simulink model "ParameterTests"  (R2019b)
settings: Solver=FixedStepAuto  StartTime=0.0  StopTime=tf  RelTol=1e-3  EnableMultiTasking=on
undefined symbols (not defined in the file or in its folder): bias
libraries: xpcrtudplib x4, slrtlib x4, xpcutilitieslib x3, speedgoatlib_IO101 x2, dspstat3 x2, dspsrcs4 x1
settings Model: SimulationMode=external  Creator=kflambet  LastModifiedBy=Sharma Lab
settings SolverCC: ConcurrentTasks=on  AutoInsertRateTranBlk=on
settings DataIOCC: SaveFormat=StructureWithTime
settings OptimizationCC: BlockReduction=off  OptimizeBlockIOStorage=off  BufferReuse=off  GlobalBufferReuse=off  ExpressionFolding=off  LocalBlockOutputs=off  OptimizeDataStoreBuffers=off  BusAssignmentInplaceUpdate=off
settings HardwareCC: ProdBitPerPointer=32  ProdBitPerSizeT=32  ProdBitPerPtrDiffT=32  ProdLargestAtomicFloat=None  ProdWordSize=32  ProdLongLongMode=on  ProdHWDeviceType=Generic->32-bit x86 compatible
settings RTWCC: Description=Simulink Real-Time  SystemTargetFile=slrt.tlc  TemplateMakefile=slrt_default_tmf  CodeExecutionProfiling=on  RTWCompilerOptimization=on
settings SimulinkRealTimeCC: SupportVariableSizeSignals=on  PreserveStateflowLocalDataDimensions=off  RL32LogTETModifier=off  xPCConcurrentTasks=on

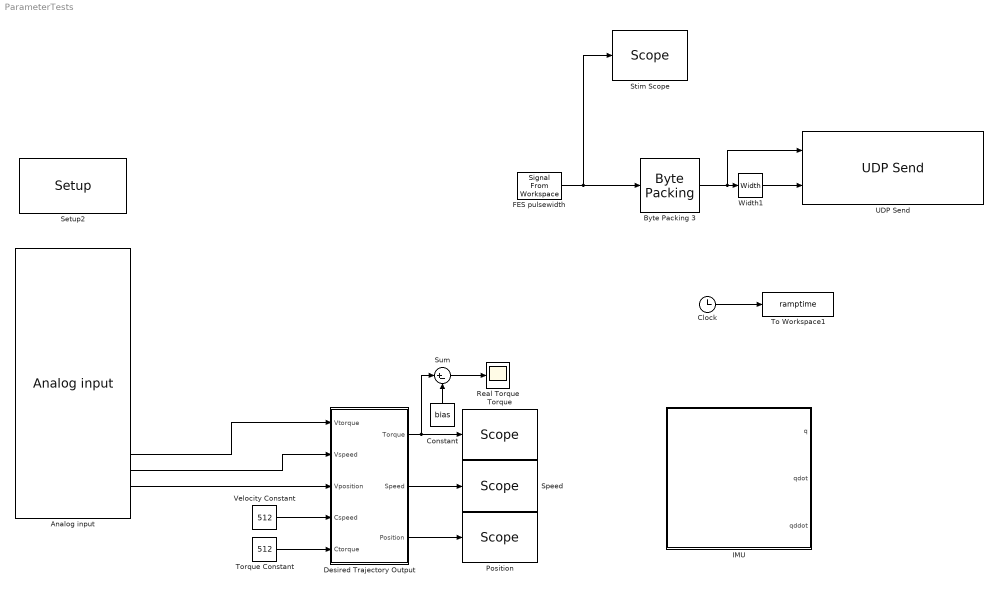
== system ParameterTests ==
  Analog input : speedgoatlib_IO101/Analog input  id=1  startChannel=1  numChannels=16  coupling=1  range=3  acqMode=1  outpMode=Values  ts=0.001  pciSlot=-1
      settings: SourceProductName=Simulink Real-Time: Speedgoat Library
  Byte Packing 3 : xpcutilitieslib/Byte Packing   MaskPackedDataType=uint8  MaskUnpackedDataTypes={ 'double'}  MaskAlignment=8
  Clock : Clock
  Constant : Constant  Value=bias
  Desired Trajectory Output : MATLAB Function  TreatAsAtomicUnit=on
  FES pulsewidth : dspsrcs4/Signal From Workspace  X=stim  Ts=0.001  nsamps=1  OutputAfterFinalValue=Setting to zero  ignoreOrWarnInputAndFrameLengths=off  OutputFrames=off
  IMU : Subsystem
  Position : slrtlib/Displays and Logging/Scope   scopeno=3  scopetype=Target  autostart=on  viewmode=Graphical sliding  formatstr='%15.6f'  grid=on  ylimits=[-360 360]  nosamples=10000  noprepostsamples=0  interleave=1  triggermode=FreeRun  triggersignal=1  trigsignalfromport=off  triggerlevel=0.0  triggerslope=Either  triggerscope=1  triggersample=0  filename=data.dat  mode=Lazy  writesize=512  autorestart=off  dynamicfilemode=off  maxwritefilesize=512*1024^2
  Real Torque : Scope
  Setup2 : speedgoatlib_IO101/Setup  group=Analog input setup  id=1  pciSlot=-1  adStartChannel=1  adNumChannel=16  adCoupling=Differential  adRange="-10 .. 10V ==> Set  hardware DIP switches 2 5 6 9 to ON"  adAcqMode=Standard  daChannel=[1:8]  daReset=[1]  daInitValue=[0]  lowerChannel=1  lowerDirection=Input  lowerDIDebounce=0  lowerDOReset=[1]  lowerDOInitValues=[0]  upperChannel=1  upperDirection=Output  upperDIDebounce=0  upperDOReset=0  upperDOInitValues=0
      settings: SourceProductName=Simulink Real-Time: Speedgoat Library
  Speed : slrtlib/Displays and Logging/Scope   scopeno=5  scopetype=Target  autostart=on  viewmode=Graphical sliding  formatstr='%15.6f'  grid=on  ylimits=[-64 64]  nosamples=10000  noprepostsamples=0  interleave=1  triggermode=FreeRun  triggersignal=1  trigsignalfromport=off  triggerlevel=0.0  triggerslope=Either  triggerscope=1  triggersample=0  filename=data.dat  mode=Lazy  writesize=512  autorestart=off  dynamicfilemode=off  maxwritefilesize=512*1024^2
  Stim Scope : slrtlib/Displays and Logging/Scope   scopeno=2  scopetype=Target  autostart=on  viewmode=Graphical sliding  formatstr='%15.6f'  grid=on  ylimits=[0,50]  nosamples=2000  noprepostsamples=0  interleave=1  triggermode=FreeRun  triggersignal=1  trigsignalfromport=off  triggerlevel=0.0  triggerslope=Either  triggerscope=1  triggersample=0  filename=data.dat  mode=Lazy  writesize=512  autorestart=off  dynamicfilemode=off  maxwritefilesize=512*1024^2
  Sum : Sum  Inputs=|+-
  To Workspace1 : ToWorkspace  VariableName=ramptime  SaveFormat=Timeseries  SampleTime=-1
  Torque : slrtlib/Displays and Logging/Scope   scopeno=1  scopetype=Target  autostart=on  viewmode=Graphical sliding  formatstr='%15.6f'  grid=on  ylimits=[-128 128]  nosamples=10000  noprepostsamples=0  interleave=1  triggermode=FreeRun  triggersignal=1  trigsignalfromport=off  triggerlevel=0.0  triggerslope=Either  triggerscope=1  triggersample=0  filename=data.dat  mode=Lazy  writesize=512  autorestart=off  dynamicfilemode=off  maxwritefilesize=512*1024^2
  Torque Constant : Constant  Value=512
  UDP Send : xpcrtudplib/UDP Send  ipAddressVal=192.168.1.2  localPort=25001  toAddress=255.255.255.255  toPort=8001  sampleTime=.05
      settings: SourceProductName=Simulink Real-Time  SourceProductBaseCode=XP
  Velocity Constant : Constant  Value=512
  Width1 : Width
  wires:
  Width1/1 -> UDP Send/2
  Byte Packing 3/1 -> UDP Send/1, Width1/1
  FES pulsewidth/1 -> Byte Packing 3/1, Stim Scope/1
  Clock/1 -> To Workspace1/1
  Desired Trajectory Output/2(Speed) -> Speed/1
  Desired Trajectory Output/1(Torque) -> Sum/1, Torque/1
  Analog input/14 -> Desired Trajectory Output/2(Vspeed)
  Analog input/13 -> Desired Trajectory Output/1(Vtorque)
  Desired Trajectory Output/3(Position) -> Position/1
  Analog input/15 -> Desired Trajectory Output/3(Vposition)
  Velocity Constant/1 -> Desired Trajectory Output/4(Cspeed)
  Torque Constant/1 -> Desired Trajectory Output/5(Ctorque)
  Constant/1 -> Sum/2
  Sum/1 -> Real Torque/1

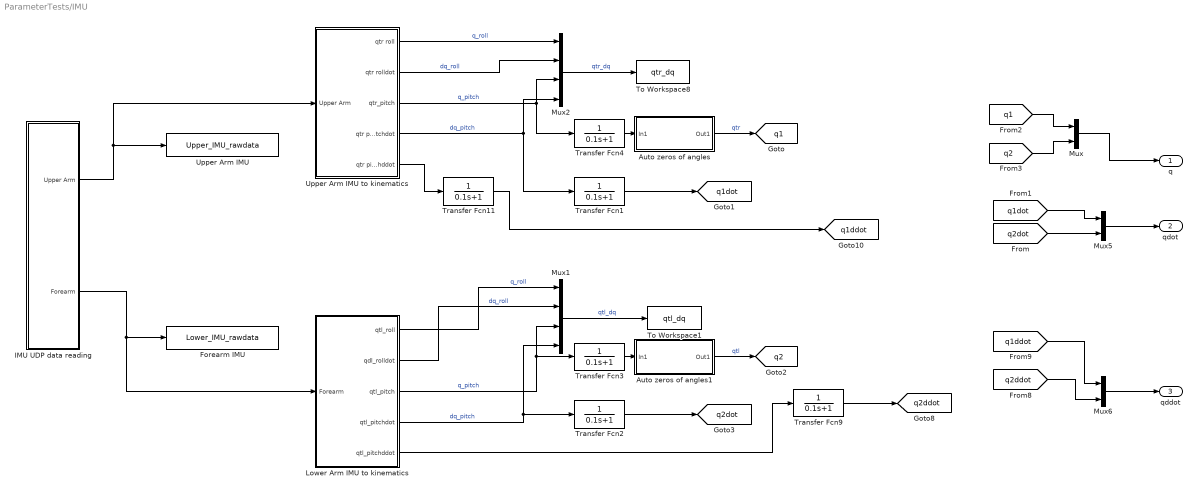
== system ParameterTests/IMU ==
  Auto zeros of angles : Subsystem
  Auto zeros of angles1 : Subsystem
  Forearm IMU : ToWorkspace  VariableName=Lower_IMU_rawdata  SampleTime=-1
  IMU UDP data reading : Subsystem
  Lower Arm IMU to kinematics : Subsystem
  Mux : Mux  Inputs=2
  Mux1 : Mux
  Mux2 : Mux
  Mux5 : Mux  Inputs=2
  Mux6 : Mux  Inputs=2
  To Workspace1 : ToWorkspace  VariableName=qtl_dq  SaveFormat=Structure With Time  SampleTime=-1
      settings: Save2DSignal=2-D array (concatenate along first dimension)
  To Workspace8 : ToWorkspace  VariableName=qtr_dq  SaveFormat=Structure With Time  SampleTime=-1
      settings: Save2DSignal=2-D array (concatenate along first dimension)
  Transfer Fcn{1..4,9,11} (6 alike) : TransferFcn  Numerator=[0 1]  Denominator=[0.1 1]
  Upper Arm IMU : ToWorkspace  VariableName=Upper_IMU_rawdata  SampleTime=-1
  Upper Arm IMU to kinematics : Subsystem
  q : Outport
  qdot : Outport  Port=2
  qddot : Outport  Port=3
  tag scope: q1=global, q1ddot=global, q1dot=global, q2=global, q2ddot=global, q2dot=global
  wires:
  IMU UDP data reading/1(Upper Arm) -> Upper Arm IMU/1, Upper Arm IMU to kinematics/1(Upper Arm)
  IMU UDP data reading/2(Forearm) -> Lower Arm IMU to kinematics/1(Forearm), Forearm IMU/1
  Transfer Fcn1/1 -> [q1dot]
  Upper Arm IMU to kinematics/4(qtr pitchdot) -> Transfer Fcn1/1, Mux2/4  "dq_pitch"
  Transfer Fcn4/1 -> Auto zeros of angles/1(In1)
  Upper Arm IMU to kinematics/3(qtr_pitch) -> Transfer Fcn4/1, Mux2/3  "q_pitch"
  Upper Arm IMU to kinematics/1(qtr roll) -> Mux2/1  "q_roll"
  Auto zeros of angles/1(Out1) -> [q1]  "qtr"
  Upper Arm IMU to kinematics/2(qtr rolldot) -> Mux2/2  "dq_roll"
  Mux2/1 -> To Workspace8/1  "qtr_dq"
  Auto zeros of angles1/1(Out1) -> [q2]  "qtl"
  Transfer Fcn3/1 -> Auto zeros of angles1/1(In1)
  Lower Arm IMU to kinematics/4(qtl_pitchdot) -> Mux1/4, Transfer Fcn2/1  "dq_pitch"
  Lower Arm IMU to kinematics/2(qdl_rolldot) -> Mux1/2  "dq_roll"
  Transfer Fcn2/1 -> [q2dot]
  Mux1/1 -> To Workspace1/1  "qtl_dq"
  Lower Arm IMU to kinematics/1(qtl_roll) -> Mux1/1  "q_roll"
  Lower Arm IMU to kinematics/3(qtl_pitch) -> Mux1/3, Transfer Fcn3/1  "q_pitch"
  Lower Arm IMU to kinematics/5(qtl_pitchddot) -> Transfer Fcn9/1
  Transfer Fcn9/1 -> [q2ddot]
  Upper Arm IMU to kinematics/5(qtr pitchddot) -> Transfer Fcn11/1
  Transfer Fcn11/1 -> [q1ddot]
  [q2dot] -> Mux5/2
  [q1dot] -> Mux5/1
  [q1ddot] -> Mux6/1
  [q2ddot] -> Mux6/2
  Mux5/1 -> qdot/1
  Mux6/1 -> qddot/1
  Mux/1 -> q/1
  [q1] -> Mux/1
  [q2] -> Mux/2

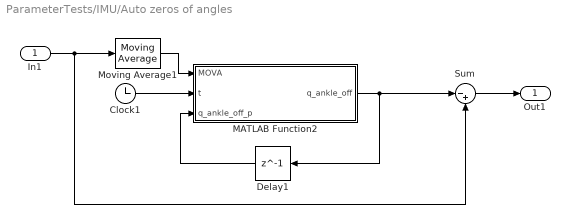
== system ParameterTests/IMU/Auto zeros of angles ==
  In1 : Inport
  Clock1 : Clock
  Delay1 : Delay  DelayLength=1  InitialCondition=1
  MATLAB Function2 : MATLAB Function  TreatAsAtomicUnit=on
  Moving Average1 : dspstat3/Moving Average  Method=Sliding window  ForgettingFactorPort=off  SpecifyWindowLength=on  WindowLength=500  ForgettingFactor=0.9  SimulateUsing=Code generation
  Sum : Sum  Inputs=|-+
  Out1 : Outport
  wires:
  MATLAB Function2/1(q_ankle_off) -> Sum/1, Delay1/1
  Clock1/1 -> MATLAB Function2/2(t)
  Delay1/1 -> MATLAB Function2/3(q_ankle_off_p)
  Moving Average1/1 -> MATLAB Function2/1(MOVA)
  In1/1 -> Sum/2, Moving Average1/1
  Sum/1 -> Out1/1

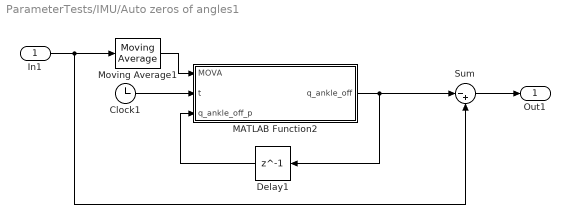
== system ParameterTests/IMU/Auto zeros of angles1 ==
  In1 : Inport
  Clock1 : Clock
  Delay1 : Delay  DelayLength=1  InitialCondition=1
  MATLAB Function2 : MATLAB Function  TreatAsAtomicUnit=on
  Moving Average1 : dspstat3/Moving Average  Method=Sliding window  ForgettingFactorPort=off  SpecifyWindowLength=on  WindowLength=500  ForgettingFactor=0.9  SimulateUsing=Code generation
  Sum : Sum  Inputs=|-+
  Out1 : Outport
  wires:
  MATLAB Function2/1(q_ankle_off) -> Sum/1, Delay1/1
  Clock1/1 -> MATLAB Function2/2(t)
  Delay1/1 -> MATLAB Function2/3(q_ankle_off_p)
  Moving Average1/1 -> MATLAB Function2/1(MOVA)
  In1/1 -> Sum/2, Moving Average1/1
  Sum/1 -> Out1/1

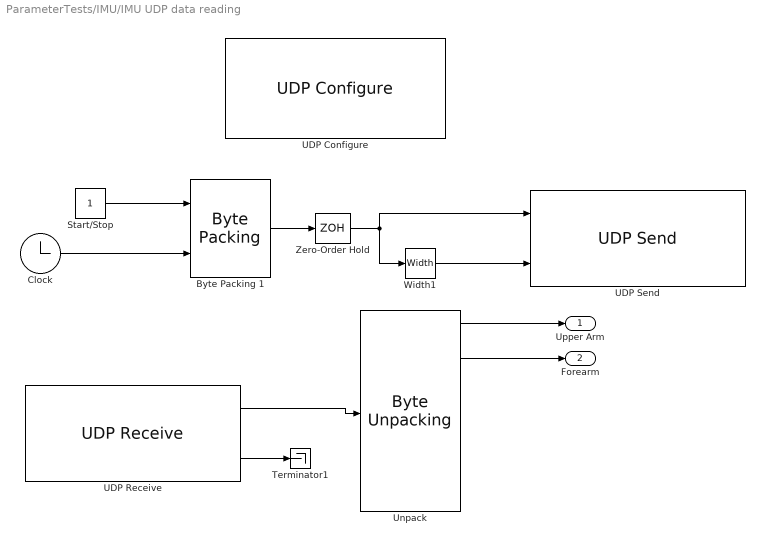
== system ParameterTests/IMU/IMU UDP data reading ==
  Byte Packing 1 : xpcutilitieslib/Byte Packing   MaskPackedDataType=uint8  MaskUnpackedDataTypes={'boolean', 'double'}  MaskAlignment=8
  Clock : Clock
      settings: Decimation=20
  Start/Stop : Constant  OutDataTypeStr=boolean
  Terminator1 : Terminator
  UDP Configure : xpcrtudplib/UDP Configure  Priority=-1  IpAddress=192.168.1.2  SubnetMask=255.255.255.0  Gateway=192.168.1.1  PciBus=2  PciSlot=0  PciFunction=0  ID=1  tune=0  disable=off  enableMulticast=off  MulticastIpAddress={}  MulticastMask={}
      settings: SourceProductBaseCode=XP
  UDP Receive : xpcrtudplib/UDP Receive  ipAddressVal=192.168.1.2  localPort=10000  rcvWidth=288  rcvFmAny=off  fmAddress=0.0.0.0  rcvMulticast=off  multicastAddress={}  maxUDPQueue=8  sampleTime=0.001
  UDP Send : xpcrtudplib/UDP Send  ipAddressVal=192.168.1.2  localPort=10000  toAddress=255.255.255.255  toPort=10000  sampleTime=-1
      settings: SourceProductBaseCode=XP
  Unpack : xpcutilitieslib/Byte Unpacking   MaskUnpackedDataTypes={['double'],['double'],['double'],['double'],['double'],['double']}  MaskUnpackedDataSizes={[6],[6],[6],[6],[6],[6]}  MaskAlignment=8
      settings: SourceProductBaseCode=XP
  Width1 : Width
  Zero-Order Hold : ZeroOrderHold  SampleTime=0.001
  Upper Arm : Outport
  Forearm : Outport  Port=2
  wires:
  Start/Stop/1 -> Byte Packing 1/1
  Byte Packing 1/1 -> Zero-Order Hold/1
  Unpack/2 -> Forearm/1
  Unpack/1 -> Upper Arm/1
  UDP Receive/2 -> Terminator1/1
  Width1/1 -> UDP Send/2
  Zero-Order Hold/1 -> UDP Send/1, Width1/1
  UDP Receive/1 -> Unpack/1
  Clock/1 -> Byte Packing 1/2

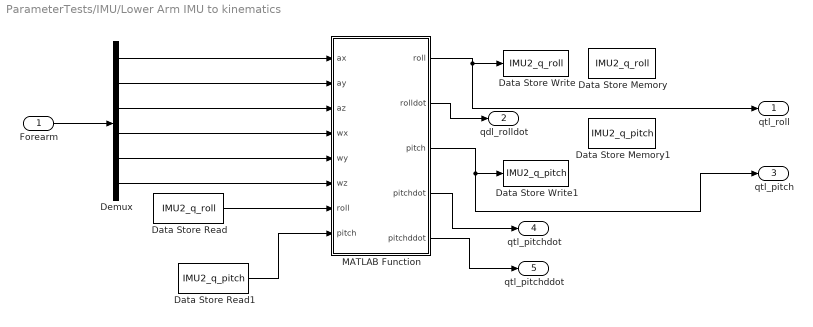
== system ParameterTests/IMU/Lower Arm IMU to kinematics ==
  Forearm : Inport
  Data Store Memory : DataStoreMemory  DataStoreName=IMU2_q_roll  ReadBeforeWriteMsg=warning  WriteAfterWriteMsg=warning  WriteAfterReadMsg=warning  ShowAdditionalParam=off
  Data Store Memory1 : DataStoreMemory  DataStoreName=IMU2_q_pitch  ReadBeforeWriteMsg=warning  WriteAfterWriteMsg=warning  WriteAfterReadMsg=warning  ShowAdditionalParam=off
  Data Store Read : DataStoreRead  DataStoreName=IMU2_q_roll
  Data Store Read1 : DataStoreRead  DataStoreName=IMU2_q_pitch
  Data Store Write : DataStoreWrite  DataStoreName=IMU2_q_roll
  Data Store Write1 : DataStoreWrite  DataStoreName=IMU2_q_pitch
  Demux : Demux  Outputs=6
  MATLAB Function : MATLAB Function  TreatAsAtomicUnit=on
  qtl_roll : Outport
  qdl_rolldot : Outport  Port=2
  qtl_pitch : Outport  Port=3
  qtl_pitchdot : Outport  Port=4
  qtl_pitchddot : Outport  Port=5
  wires:
  MATLAB Function/4(pitchdot) -> qtl_pitchdot/1
  MATLAB Function/2(rolldot) -> qdl_rolldot/1
  MATLAB Function/3(pitch) -> qtl_pitch/1, Data Store Write1/1
  Demux/2 -> MATLAB Function/2(ay)
  MATLAB Function/1(roll) -> qtl_roll/1, Data Store Write/1
  Demux/6 -> MATLAB Function/6(wz)
  Demux/5 -> MATLAB Function/5(wy)
  Demux/4 -> MATLAB Function/4(wx)
  Data Store Read/1 -> MATLAB Function/7("roll ")
  Demux/1 -> MATLAB Function/1(ax)
  Demux/3 -> MATLAB Function/3(az)
  Forearm/1 -> Demux/1
  Data Store Read1/1 -> MATLAB Function/8("pitch ")
  MATLAB Function/5(pitchddot) -> qtl_pitchddot/1

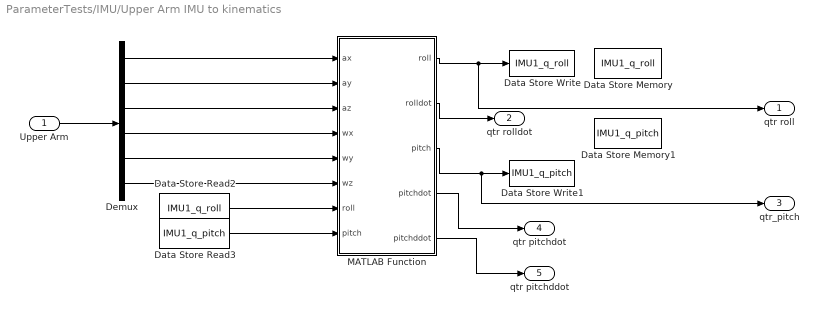
== system ParameterTests/IMU/Upper Arm IMU to kinematics ==
  Upper Arm : Inport
  Data Store Memory : DataStoreMemory  DataStoreName=IMU1_q_roll  ReadBeforeWriteMsg=warning  WriteAfterWriteMsg=warning  WriteAfterReadMsg=warning  ShowAdditionalParam=off
  Data Store Memory1 : DataStoreMemory  DataStoreName=IMU1_q_pitch  ReadBeforeWriteMsg=warning  WriteAfterWriteMsg=warning  WriteAfterReadMsg=warning  ShowAdditionalParam=off
  Data Store Read2 : DataStoreRead  DataStoreName=IMU1_q_roll
  Data Store Read3 : DataStoreRead  DataStoreName=IMU1_q_pitch
  Data Store Write : DataStoreWrite  DataStoreName=IMU1_q_roll
  Data Store Write1 : DataStoreWrite  DataStoreName=IMU1_q_pitch
  Demux : Demux  Outputs=6
  MATLAB Function : MATLAB Function  TreatAsAtomicUnit=on
  qtr roll : Outport
  qtr rolldot : Outport  Port=2
  qtr_pitch : Outport  Port=3
  qtr pitchdot : Outport  Port=4
  qtr pitchddot : Outport  Port=5
  wires:
  Upper Arm/1 -> Demux/1
  Demux/1 -> MATLAB Function/1(ax)
  Demux/2 -> MATLAB Function/2(ay)
  Demux/3 -> MATLAB Function/3(az)
  Demux/4 -> MATLAB Function/4(wx)
  Demux/5 -> MATLAB Function/5(wy)
  Demux/6 -> MATLAB Function/6(wz)
  Data Store Read2/1 -> MATLAB Function/7("roll ")
  Data Store Read3/1 -> MATLAB Function/8("pitch ")
  MATLAB Function/1(roll) -> qtr roll/1, Data Store Write/1
  MATLAB Function/3(pitch) -> Data Store Write1/1, qtr_pitch/1
  MATLAB Function/2(rolldot) -> qtr rolldot/1
  MATLAB Function/4(pitchdot) -> qtr pitchdot/1
  MATLAB Function/5(pitchddot) -> qtr pitchddot/1

== matlab function ParameterTests/Desired Trajectory Output ==
  data: Vtorque input; Vspeed input; Torque output; Vposition input; Cspeed input; Ctorque input; Speed output; Position output
function [Torque,Speed,Position] = BiodexGain(Vtorque,Vspeed,Vposition,Cspeed,Ctorque)

%%% This function outputs the correct torque, speed, and position values
%%% from the Biodex given the raw voltage and the conversion factors
%%% (Cspeed and Ctorque).

switch Cspeed

    case 512
    Speed=Vspeed/0.0098;
       
    case 256
    Speed=Vspeed/0.0195;
       
    case 128
    Speed=Vspeed/0.0391;
      
       
    case 64
    Speed=Vspeed/0.0781;
    
    case 32
    Speed=Vspeed/0.1563; 
      
    otherwise
    Speed=-1;
    
end

switch Ctorque

    case 512
    Torque=Vtorque/0.0098;
       
    case 256
    Torque=Vtorque/0.0195;
       
    case 128
    Torque=Vtorque/0.0391;
      
       
    case 64
    Torque=Vtorque/0.0781;
    
    case 32
    Torque=Vtorque/0.1563; 
      
    otherwise
    Torque=-1;
    
end

Position = Vposition/0.0292;

end

== matlab function ParameterTests/IMU/Lower Arm IMU to kinematics/MATLAB Function ==
  data: ax input; roll output; ay input; az input; wx input; wy input; wz input; rolldot output; pitch output; pitchdot output; roll input; pitch input; pitchddot output
function [roll,rolldot,pitch,pitchdot,pitchddot] = fcn(ax,ay,az,wx,wy,wz,roll,pitch)

%%% ax, ay, az = angular accelerations
%%% wx, wy, wz = angular velocities

    Ts = 0.001; % time step [s]
    a = 0.99;
    A_roll = atan2(ay,(ax*ax+az*az)^0.5);
    A_pitch = atan2(-ax,(ay*ay+az*az)^0.5);

    G_roll = wx*Ts; rolldot = wx;
    G_pitch = wy*Ts; pitchdot = wy; pitchddot = ay;
    G_yaw = wz*Ts;
    
    roll = a*(roll+G_roll) + (1-a)*A_roll;
    pitch = a*(pitch+G_pitch) + (1-a)*A_pitch;

end

== matlab function ParameterTests/IMU/Upper Arm IMU to kinematics/MATLAB Function ==
  data: ax input; roll output; ay input; az input; wx input; wy input; wz input; rolldot output; pitch output; pitchdot output; roll input; pitch input; pitchddot output
function [roll,rolldot,pitch,pitchdot,pitchddot] = fcn(ax,ay,az,wx,wy,wz,roll,pitch)

%%% ax, ay, az = angular accelerations
%%% wx, wy, wz = angular velocities

    Ts = 0.001; % time step [s]
    a = 0.99;
    A_roll = atan2(ay,(ax*ax+az*az)^0.5);
    A_pitch = atan2(-ax,(ay*ay+az*az)^0.5);

    G_roll = wx*Ts; rolldot = wx;
    G_pitch = wy*Ts; pitchdot = wy; pitchddot = ay;
    G_yaw = wz*Ts;
    
    roll = a*(roll+G_roll) + (1-a)*A_roll;
    pitch = a*(pitch+G_pitch) + (1-a)*A_pitch;

end

== matlab function ParameterTests/IMU/Auto zeros of angles/MATLAB Function2 ==
  data: q_ankle_off output; MOVA input; t input; q_ankle_off_p input
function q_ankle_off = fcn(MOVA, t, q_ankle_off_p)

if t <= 4
    q_ankle_off = MOVA;
else
    q_ankle_off = q_ankle_off_p;
end

== matlab function ParameterTests/IMU/Auto zeros of angles1/MATLAB Function2 ==
  data: q_ankle_off output; MOVA input; t input; q_ankle_off_p input
function q_ankle_off = fcn(MOVA, t, q_ankle_off_p)

if t <= 4
    q_ankle_off = MOVA;
else
    q_ankle_off = q_ankle_off_p;
end
